simulink model "FieldOrientedController"  (R2020a)
settings: configuration reference "SLRT" (kept outside this file)
undefined symbols (not defined in the file): paramAdcAmperePerTransducerVolt, paramAdcTransducerVoltAtZeroAmpere, paramCurrentControlI, paramCurrentControlP, paramCurrentControlSatVoltage, paramEncoderCalibrationDuration, paramEncoderCalibrationMaxError, paramEncoderCalibrationVoltage, paramEncoderRotorPositionAtZeroCount, paramEncoderRotorPositionPerCount, paramOpenLoopVelocityAcceleration, paramOpenLoopVelocityToVoltsBias, paramOpenLoopVelocityToVoltsScalar, paramOverCurrentDuration, paramOverCurrentEnable, paramOverCurrentLimit, paramPwmCompareAtZeroVolt, paramPwmCompareMax, paramPwmComparePerVolt, paramVelocityControlI, paramVelocityControlP, paramVelocityControlSatCurrent, paramVelocityFilterCoeffDen, paramVelocityFilterCoeffNum, PolePairs, sampleTime
libraries: simulink x5
(part 1 of 2)
settings Model: DataDictionary=SGKitControllerData.sldd  EnableAccessToBaseWorkspace=off  OrderedModelArguments=off  Creator=The MathWorks, Inc.  LastModifiedBy=daniel.fonte
settings ConfigSetRef: SourceName=SLRT

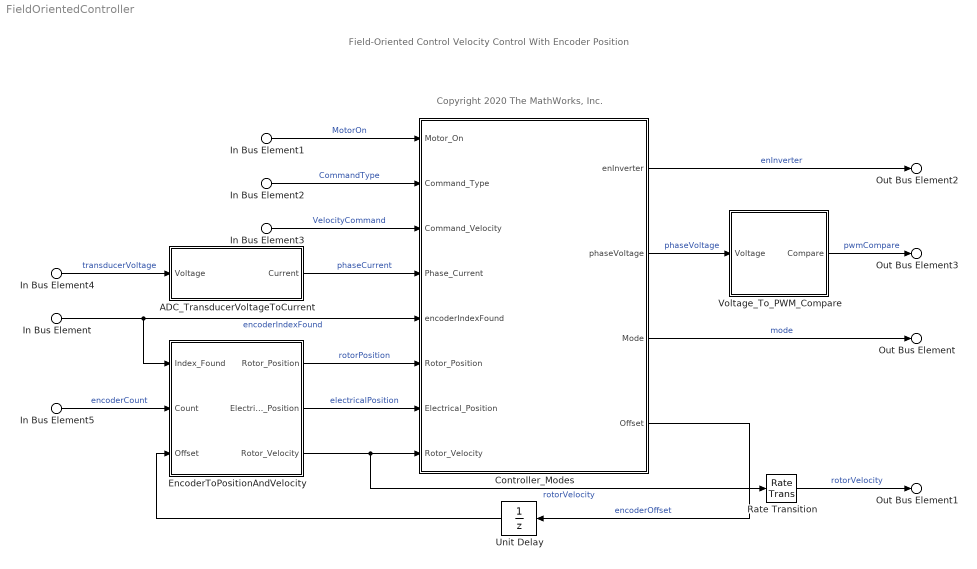
== system FieldOrientedController ==
  note: Field-Oriented Control
      | Velocity Control With Encoder Position
  note: Copyright 2020 The MathWorks, Inc.
  In Bus Element1 : Inport  PortName=userInputs  Element=motorOn
  In Bus Element2 : Inport  PortName=userInputs  Element=commandType
  In Bus Element3 : Inport  PortName=userInputs  Element=velocityCommand
  In Bus Element4 : Inport  Port=2  PortName=controllerFeedback  Element=transducerVoltage
  In Bus Element : Inport  Port=2  PortName=controllerFeedback  Element=encoderIndexFound
  In Bus Element5 : Inport  Port=2  PortName=controllerFeedback  Element=encoderCount
  ADC_TransducerVoltageToCurrent : Subsystem  VariantControl=kitType == 1
  Controller_Modes : Subsystem
  EncoderToPositionAndVelocity : Subsystem  VariantControl=ctrlVariantPosSns==PosSnsEnum.Encoder
  Rate Transition : RateTransition  OutPortSampleTime=sampleTime.VelocityControl
  Unit Delay : UnitDelay  InitialCondition=paramEncoderRotorPositionAtZeroCount  SampleTime=-1  StateName=encoderOffset  HasFrameUpgradeWarning=on
  Voltage_To_PWM_Compare : Subsystem
  Out Bus Element : Outport  PortName=controllerInfo  Element=mode
  Out Bus Element1 : Outport  PortName=controllerInfo  Element=rotorVelocity
  Out Bus Element2 : Outport  Port=2  PortName=motorCommands  Element=enInverter
  Out Bus Element3 : Outport  Port=2  PortName=motorCommands  Element=pwmCompare
  wires:
  EncoderToPositionAndVelocity/2(Electrical_Position) -> Controller_Modes/7(Electrical_Position)  "electricalPosition"
  EncoderToPositionAndVelocity/3(Rotor_Velocity) -> Rate Transition/1, Controller_Modes/8(Rotor_Velocity)  "rotorVelocity"
  Controller_Modes/4(Offset) -> Unit Delay/1  "encoderOffset"
  EncoderToPositionAndVelocity/1(Rotor_Position) -> Controller_Modes/6(Rotor_Position)  "rotorPosition"
  In Bus Element1/1 -> Controller_Modes/1(Motor_On)  "MotorOn"
  In Bus Element2/1 -> Controller_Modes/2(Command_Type)  "CommandType"
  In Bus Element3/1 -> Controller_Modes/3(Command_Velocity)  "VelocityCommand"
  In Bus Element/1 -> Controller_Modes/5(encoderIndexFound), EncoderToPositionAndVelocity/1(Index_Found)  "encoderIndexFound"
  Voltage_To_PWM_Compare/1(Compare) -> Out Bus Element3/1  "pwmCompare"
  In Bus Element5/1 -> EncoderToPositionAndVelocity/2(Count)  "encoderCount"
  Unit Delay/1 -> EncoderToPositionAndVelocity/3(Offset)
  In Bus Element4/1 -> ADC_TransducerVoltageToCurrent/1(Voltage)  "transducerVoltage"
  ADC_TransducerVoltageToCurrent/1(Current) -> Controller_Modes/4(Phase_Current)  "phaseCurrent"
  Controller_Modes/1(enInverter) -> Out Bus Element2/1  "enInverter"
  Controller_Modes/2(phaseVoltage) -> Voltage_To_PWM_Compare/1(Voltage)  "phaseVoltage"
  Controller_Modes/3(Mode) -> Out Bus Element/1  "mode"
  Rate Transition/1 -> Out Bus Element1/1  "rotorVelocity"

== system FieldOrientedController/ADC_TransducerVoltageToCurrent ==
  note: ADC Transducer Voltage to Current
  Voltage : Inport
  Add : Sum  Inputs=+-
  Bias_To_Remove : Constant  Value=paramAdcTransducerVoltAtZeroAmpere  OutDataTypeStr=Inherit: Inherit via back propagation  SampleTime=-1
  Product : Product
  Scalar : Constant  Value=paramAdcAmperePerTransducerVolt  OutDataTypeStr=Inherit: Inherit via back propagation  SampleTime=-1
  Current : Outport  VectorParamsAs1DForOutWhenUnconnected=off
  wires:
  Voltage/1 -> Add/1
  Scalar/1 -> Product/2
  Add/1 -> Product/1
  Bias_To_Remove/1 -> Add/2
  Product/1 -> Current/1  "PhaseCurrent"

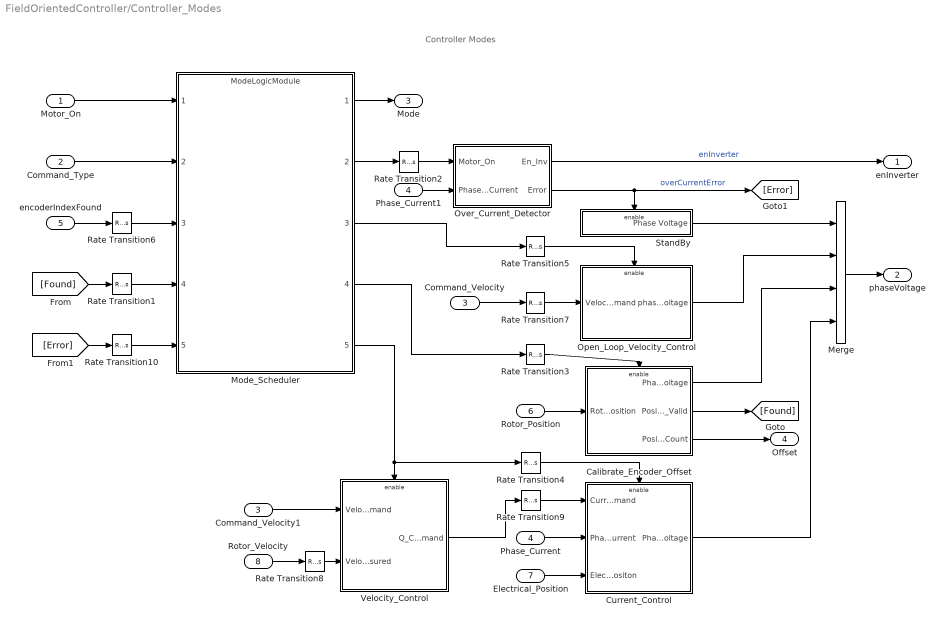
== system FieldOrientedController/Controller_Modes ==
  note: Controller Modes
  Motor_On : Inport
  Command_Type : Inport  Port=2
  Command_Velocity : Inport  Port=3
  Phase_Current : Inport  Port=4
  encoderIndexFound : Inport  Port=5
  Rotor_Position : Inport  Port=6
  Electrical_Position : Inport  Port=7
  Rotor_Velocity : Inport  Port=8
  Calibrate_Encoder_Offset : Subsystem
      mask Display: fprintf('Calibrate\nEncoder\nOffset')
  Command_Velocity1 : InportShadow  Port=3
  Current_Control : Subsystem
      mask Display: fprintf('Current\nControl')
  Merge : Merge  Inputs=4
      mask Display: fprintf(' ')
  Mode_Scheduler : ModelReference  ModelNameDialog=ModeLogicModule  SimulationMode=Normal  ModelReferenceVersion=1.378
  Open_Loop_Velocity_Control : Subsystem  TreatAsAtomicUnit=on
      settings: RTWFcnNameOpts=User specified  FunctionInterfaceSpec=Allow arguments (Optimized)
      mask Display: fprintf('Open Loop\nVelocity\nControl')
  Over_Current_Detector : Subsystem
      mask Display: %fprintf('Detect\nOvercurrent')
  Phase_Current1 : InportShadow  Port=4
  Rate Transition{1,6,8,10} (4 alike) : RateTransition  Integrity=off  OutPortSampleTime=sampleTime.VelocityControl
  Rate Transition{2..5,9} (5 alike) : RateTransition  Integrity=off
  Rate Transition7 : RateTransition  Integrity=off  OutPortSampleTime=sampleTime.CurrentControl
  StandBy : Subsystem  Description=Stand By mode for controller outputs constant phase voltages.  TreatAsAtomicUnit=on
      mask Display: fprintf('Disabled')
  Velocity_Control : Subsystem
      mask Display: fprintf('Velocity\nControl')
  enInverter : Outport  VectorParamsAs1DForOutWhenUnconnected=off
  phaseVoltage : Outport  Port=2  VectorParamsAs1DForOutWhenUnconnected=off
  Mode : Outport  Port=3  VectorParamsAs1DForOutWhenUnconnected=off
  Offset : Outport  Port=4  VectorParamsAs1DForOutWhenUnconnected=off
  wires:
  Rate Transition10/1 -> Mode_Scheduler/5
  [Error] -> Rate Transition10/1
  Calibrate_Encoder_Offset/2(Position_At_Zero_Count_Valid) -> [Found]
  Over_Current_Detector/2(Error) -> [Error], StandBy/Enable  "overCurrentError"
  Phase_Current1/1 -> Over_Current_Detector/2(Phase_Current)
  Rate Transition2/1 -> Over_Current_Detector/1(Motor_On)
  Mode_Scheduler/2 -> Rate Transition2/1
  Motor_On/1 -> Mode_Scheduler/1
  [Found] -> Rate Transition1/1
  Merge/1 -> phaseVoltage/1
  Command_Velocity/1 -> Rate Transition7/1
  Calibrate_Encoder_Offset/3(Position_At_Zero_Count) -> Offset/1
  Rotor_Position/1 -> Calibrate_Encoder_Offset/1(Rotor_Position)
  Calibrate_Encoder_Offset/1(Phase_Voltage) -> Merge/3
  StandBy/1(Phase Voltage) -> Merge/1
  Command_Type/1 -> Mode_Scheduler/2
  Mode_Scheduler/1 -> Mode/1
  Mode_Scheduler/4 -> Rate Transition3/1
  Rate Transition3/1 -> Calibrate_Encoder_Offset/Enable
  Rate Transition1/1 -> Mode_Scheduler/4
  Rate Transition7/1 -> Open_Loop_Velocity_Control/1(Velocity_Command)
  Open_Loop_Velocity_Control/1(phase_voltage) -> Merge/2
  Current_Control/1(Phase_Voltage) -> Merge/4
  Rate Transition4/1 -> Current_Control/Enable
  Rate Transition9/1 -> Current_Control/1(Current_Command)
  Velocity_Control/1(Q_Current_Command) -> Rate Transition9/1
  Mode_Scheduler/5 -> Rate Transition4/1, Velocity_Control/Enable
  Phase_Current/1 -> Current_Control/2(Phase_Current)
  Electrical_Position/1 -> Current_Control/3(Electrical_Positon)
  Rotor_Velocity/1 -> Rate Transition8/1
  Command_Velocity1/1 -> Velocity_Control/1(Velocity_Command)
  Rate Transition5/1 -> Open_Loop_Velocity_Control/Enable
  Mode_Scheduler/3 -> Rate Transition5/1
  encoderIndexFound/1 -> Rate Transition6/1
  Rate Transition8/1 -> Velocity_Control/2(Velocity_Measured)
  Over_Current_Detector/1(En_Inv) -> enInverter/1  "enInverter"
  Rate Transition6/1 -> Mode_Scheduler/3

== system FieldOrientedController/EncoderToPositionAndVelocity ==
  note: Quadrature Encoder To Position And Velocity
  Index_Found : Inport
  Count : Inport  Port=2
  Offset : Inport  Port=3
  Encoder_Count_To_Rotor_Position : Subsystem
  FilterTs15mS : DiscreteFilter  Numerator=paramVelocityFilterCoeffNum  Denominator=paramVelocityFilterCoeffDen  SampleTime=sampleTime.CurrentControl
  Position_Delta_To_Velocity : Subsystem  mask(Rotor position delta to velocity){positionDeltaBufferLength=8, sampleFrequency=1/sampleTime.EncoderPosition}
      mask prompts: positionDeltaBufferLength "Delay buffer length (must be power of two)"; sampleFrequency "Sample frequency (Hz)"
      mask help: Calculates velocity by summing the current position delta and a buffer of previous position deltas. Previous position deltas are stored in a circular buffer.
  Rotor_Position_Delta : Subsystem
  Rotor_To_Electrical_Position : Subsystem
      mask Display:
      | text(0.5, 0.5,...
      |   'E = mod(R*N_P_P,2\pi)',...
      |   'HorizontalAlignment', 'Center',...
      |   'VerticalAlignment', 'Middle',...
      |   'texmode', 'on')
  Rotor_Position : Outport  VectorParamsAs1DForOutWhenUnconnected=off
  Electrical_Position : Outport  Port=2  VectorParamsAs1DForOutWhenUnconnected=off
  Rotor_Velocity : Outport  Port=3  VectorParamsAs1DForOutWhenUnconnected=off
  wires:
  Rotor_Position_Delta/1(Position_Delta) -> Position_Delta_To_Velocity/1(Position_Delta)  "rotorPositionDelta"
  Offset/1 -> Encoder_Count_To_Rotor_Position/2(Position_At_Zero_Count), Rotor_Position_Delta/2(Encoder_Offset)
  Encoder_Count_To_Rotor_Position/1(Position) -> Rotor_Position_Delta/1(Rotor_Position), Rotor_To_Electrical_Position/1(R), Rotor_Position/1
  Rotor_To_Electrical_Position/1(E) -> Electrical_Position/1
  Count/1 -> Encoder_Count_To_Rotor_Position/1(Count)
  Index_Found/1 -> Rotor_Position_Delta/3(Encoder_Index_Found)
  Position_Delta_To_Velocity/1(Velocity) -> FilterTs15mS/1
  FilterTs15mS/1 -> Rotor_Velocity/1

== system FieldOrientedController/Voltage_To_PWM_Compare ==
  note: Voltage To PWM Compare
  Voltage : Inport
  Add : Sum  OutDataTypeStr=Inherit: Inherit via back propagation
  Bias : Constant  Value=paramPwmCompareAtZeroVolt  OutDataTypeStr=Inherit: Inherit via back propagation  SampleTime=-1
  Data_Type_Conversion : DataTypeConversion  OutDataTypeStr=uint16  LockScale=on
  Saturation : Saturate  UpperLimit=paramPwmCompareMax  LowerLimit=0
      settings: AttributesFormatString=|
      | --------------------------------
      | Upper Limit = %<UpperLimit>
      | Lower Limit = %<LowerLimit>
  Slope : Gain  Gain=paramPwmComparePerVolt
      settings: AttributesFormatString=|
      | ----------------------------------------
      | Gain = %<Gain>
  Compare : Outport  VectorParamsAs1DForOutWhenUnconnected=off
  wires:
  Add/1 -> Saturation/1
  Bias/1 -> Add/2
  Saturation/1 -> Data_Type_Conversion/1
  Slope/1 -> Add/1
  Voltage/1 -> Slope/1  "phaseVoltage"
  Data_Type_Conversion/1 -> Compare/1  "pwmCompare"

== system FieldOrientedController/Controller_Modes/Calibrate_Encoder_Offset ==
  note: Calibrate Encoder Offset
  Rotor_Position : Inport  PortDimensions=1  Interpolate=off
  Enable : EnablePort  StatesWhenEnabling=reset
      settings: AttributesFormatString=|
      | ----------------------------------------
      | States when enabling = %<StatesWhenEnabling>
  Encoder_Calibration : Subsystem
  Phase_Voltage : Outport  PortDimensions=3  InitialOutput=0  VectorParamsAs1DForOutWhenUnconnected=off
  Position_At_Zero_Count_Valid : Outport  Port=2  InitialOutput=0  VectorParamsAs1DForOutWhenUnconnected=off
  Position_At_Zero_Count : Outport  Port=3  InitialOutput=paramEncoderRotorPositionAtZeroCount  VectorParamsAs1DForOutWhenUnconnected=off
      settings: AttributesFormatString=|
      | ---------------------------------
      | Initial Output = %<InitialOutput>
  wires:
  Encoder_Calibration/2(Position_Valid) -> Position_At_Zero_Count_Valid/1
  Encoder_Calibration/1(Phase_Voltage) -> Phase_Voltage/1
  Rotor_Position/1 -> Encoder_Calibration/1(Rotor_Position)
  Encoder_Calibration/3(Position_At_Zero_Count) -> Position_At_Zero_Count/1

== system FieldOrientedController/Controller_Modes/Current_Control ==
  note: Current Control
  Current_Command : Inport
  Phase_Current : Inport  Port=2
  Electrical_Positon : Inport  Port=3
  Enable : EnablePort  StatesWhenEnabling=reset
      settings: AttributesFormatString=|
      | ----------------------------------------
      | States when enabling = %<StatesWhenEnabling>
  FOC_Current_Control : Subsystem
  Phase_Voltage : Outport  VectorParamsAs1DForOutWhenUnconnected=off
  wires:
  Electrical_Positon/1 -> FOC_Current_Control/3(Electrical_Position)
  FOC_Current_Control/1(Phase_Voltage) -> Phase_Voltage/1
  Current_Command/1 -> FOC_Current_Control/1(Current_Command)
  Phase_Current/1 -> FOC_Current_Control/2(Phase_Current)

== system FieldOrientedController/Controller_Modes/Open_Loop_Velocity_Control ==
  note: Open Loop Velocity Control
  Velocity_Command : Inport
  Enable : EnablePort  StatesWhenEnabling=reset
      settings: AttributesFormatString=|
      | ----------------------------------------
      | States when enabling = %<StatesWhenEnabling>
  Open_Loop_Velocity_Control : Subsystem
  Signal Conversion : SignalConversion  OverrideOpt=off
  phase_voltage : Outport  VectorParamsAs1DForOutWhenUnconnected=off
  wires:
  Open_Loop_Velocity_Control/1(Phase_Voltage) -> Signal Conversion/1  "phaseVoltage"
  Velocity_Command/1 -> Open_Loop_Velocity_Control/1(Velocity_Command)
  Signal Conversion/1 -> phase_voltage/1

== system FieldOrientedController/Controller_Modes/Over_Current_Detector ==
  note: Over Current Detector
  Motor_On : Inport
  Phase_Current : Inport  Port=2
  AND : Logic  IconShape=distinctive  AllPortsSameDT=off  OutDataTypeStr=boolean
  AND1 : Logic  IconShape=distinctive  AllPortsSameDT=off  OutDataTypeStr=boolean
  Abs : Abs
  Demux : Demux  Outputs=2
  Detect_Over_Current_Error : Stateflow chart  TreatAsAtomicUnit=on
  Enable_Over_Current_Detection : Constant  Value=paramOverCurrentEnable  OutDataTypeStr=Inherit: Inherit via back propagation
  Motor_On1 : InportShadow
  NOT : Logic  Operator=NOT  IconShape=distinctive  AllPortsSameDT=off  OutDataTypeStr=boolean
  En_Inv : Outport  VectorParamsAs1DForOutWhenUnconnected=off
  Error : Outport  Port=2  VectorParamsAs1DForOutWhenUnconnected=off
  wires:
  Enable_Over_Current_Detection/1 -> AND/2
  AND/1 -> Detect_Over_Current_Error/1(enableOverCurrentDetect)
  Motor_On1/1 -> AND1/1
  NOT/1 -> AND1/2
  AND1/1 -> En_Inv/1  "enableInverter"
  Motor_On/1 -> AND/1
  Demux/1 -> Detect_Over_Current_Error/2(phaseCurrentA)
  Detect_Over_Current_Error/1(error) -> NOT/1, Error/1  "overCurrentErrorDetected"
  Demux/2 -> Detect_Over_Current_Error/3(phaseCurrentB)
  Abs/1 -> Demux/1
  Phase_Current/1 -> Abs/1

== system FieldOrientedController/Controller_Modes/StandBy ==
  note: Disabled
  Enable : EnablePort
      settings: AttributesFormatString=|
      | ----------------------------------------
      | States when enabling = %<StatesWhenEnabling>
  Constant : Constant  Value=[0 0 0]  OutDataTypeStr=Inherit: Inherit via back propagation
  Phase Voltage : Outport  InitialOutput=[0 0 0]  VectorParamsAs1DForOutWhenUnconnected=off
      settings: AttributesFormatString=--------------------------------------------\nInitial Output = %<InitialOutput>
  wires:
  Constant/1 -> Phase Voltage/1

== system FieldOrientedController/Controller_Modes/Velocity_Control ==
  note: Velocity Control
  Velocity_Command : Inport
  Velocity_Measured : Inport  Port=2
  Enable : EnablePort  StatesWhenEnabling=reset
      settings: AttributesFormatString=|
      | ----------------------------------------
      | States when enabling = %<StatesWhenEnabling>
  Subtract : Sum  Inputs=+-
  Velocity_PID_Controller : simulink/Continuous/PID Controller  Controller=PI  Form=Parallel  TimeDomain=Discrete-time  UseExternalTs=off  SampleTime=sampleTime.VelocityControl  IntegratorMethod=Forward Euler  FilterMethod=Forward Euler  ControllerParametersSource=internal  P=paramVelocityControlP  I=paramVelocityControlI  D=0  UseFilter=on  N=0  TunerSelectOption=Transfer Function Based (PID Tuner App)  InitialConditionSource=internal  InitialConditionForIntegrator=0  InitialConditionForFilter=0  DifferentiatorICPrevScaledInput=0  ExternalReset=none  TrackingMode=off  Kt=1  LimitOutput=on  UpperSaturationLimit=paramVelocityControlSatCurrent  LowerSaturationLimit=-paramVelocityControlSatCurrent  LinearizeAsGain=off  AntiWindupMode=clamping  Kb=1  POutMin=[]  POutMax=[]  IOutMin=[]  IOutMax=[]  DOutMin=[]  DOutMax=[]  NOutMin=[]  NOutMax=[]  SumOutMin=[]  SumOutMax=[]  SaturationOutMin=[]  SaturationOutMax=[]  PParamMin=[]  PParamMax=[]  IParamMin=[]  IParamMax=[]  DParamMin=[]  DParamMax=[]  NParamMin=[]  NParamMax=[]  KbParamMin=[]  KbParamMax=[]  KtParamMin=[]  KtParamMax=[]  KbOutMin=[]  KbOutMax=[]  KtOutMin=[]  KtOutMax=[]  IntegratorOutMin=[]  IntegratorOutMax=[]  FilterOutMin=[]  FilterOutMax=[]  SumI1OutMin=[]  SumI1OutMax=[]  SumI2OutMin=[]  SumI2OutMax=[]  SumI3OutMin=[]  SumI3OutMax=[]  SumI4OutMin=[]  SumI4OutMax=[]  SumDOutMin=[]  SumDOutMax=[]  DifferentiatorOutMin=[]  DifferentiatorOutMax=[]  FilterDiffOutCoefMin=[]  FilterDiffOutCoefMax=[]  ReciprocalOutMin=[]  ReciprocalOutMax=[]  SumDenOutMin=[]  SumDenOutMax=[]  SumNumOutMin=[]  SumNumOutMax=[]  DivideOutMin=[]  DivideOutMax=[]  UdiffTsProdOutMin=[]  UdiffTsProdOutMax=[]  NTsProdOutMin=[]  NTsProdOutMax=[]  UintegralTsProdOutMin=[]  UintegralTsProdOutMax=[]  UngainTsProdOutMin=[]  UngainTsProdOutMax=[]  IntegratorContinuousStateAttributes=''  IntegratorStateMustResolveToSignalObject=off  IntegratorRTWStateStorageClass=Auto  FilterContinuousStateAttributes=''  FilterStateMustResolveToSignalObject=off  FilterRTWStateStorageClass=Auto  ParallelPVariant=InternalParameters  IdealPVariant=Disabled  IVariant=InternalParameters  DVariant=Disabled  IntegratorVariant=Discrete  SatVariant=Enabled  AWVariant=DiscClampingParallel  PCopyVariant=Disabled  TRVariant=Disabled  FdbkBlocksVariant=Forward  IdealPFdbkVariant=Disabled  SatFdbkVariant=Disabled  DerivativeFilterVariant=Disabled  NVariant=Disabled  NCopyVariant=Disabled_SignalSpec  FilterICVariant=Disabled  IntegratorICVariant=InternalICs  ExternalResetVariant=Disabled  TRSumVariant=Passthrough  SumFdbkVariant=Disabled  SumVariant=Sum_PI  TsampFilterVariant=InternalTs  TsampNgainVariant=Passthrough  TsampIntegralVariant=Passthrough
  Q_Current_Command : Outport  InitialOutput=0  VectorParamsAs1DForOutWhenUnconnected=off
  wires:
  Velocity_Command/1 -> Subtract/1
  Velocity_Measured/1 -> Subtract/2
  Velocity_PID_Controller/1 -> Q_Current_Command/1  "qCurrentCommand"
  Subtract/1 -> Velocity_PID_Controller/1

== system FieldOrientedController/EncoderToPositionAndVelocity/Encoder_Count_To_Rotor_Position ==
  note: Encoder Count To Rotor Position
  Count : Inport
  Position_At_Zero_Count : Inport  Port=2
  Add : Sum  AccumDataTypeStr=single
  Data_Type_Convert : DataTypeConversion  OutDataTypeStr=single
  Mod_Two_Pi_Once : Subsystem
      mask Display:
      | text(0.5, 0.5,'Mod 2\pi',...
      |   'HorizontalAlignment', 'Center',...
      |   'VerticalAlignment', 'Middle',...
      |   'texmode', 'on')
  Rotor_Position_Per_Count : Gain  Gain=paramEncoderRotorPositionPerCount  ParamDataTypeStr=single  OutDataTypeStr=single
      settings: AttributesFormatString=|
      | ------------------------------------------------
      | Gain = %<Gain>
  Position : Outport  VectorParamsAs1DForOutWhenUnconnected=off
  wires:
  Count/1 -> Data_Type_Convert/1
  Mod_Two_Pi_Once/1(Mod_X_Two_Pi) -> Position/1  "rotorPosition"
  Add/1 -> Mod_Two_Pi_Once/1(X)
  Rotor_Position_Per_Count/1 -> Add/1
  Position_At_Zero_Count/1 -> Add/2
  Data_Type_Convert/1 -> Rotor_Position_Per_Count/1

== system FieldOrientedController/EncoderToPositionAndVelocity/Position_Delta_To_Velocity ==
  note: Rotor Position Delta To Velocity
  Position_Delta : Inport  SampleTime=sampleTime.EncoderPosition
  Rotor_Position_Delta_To_Velocity : MATLAB Function  TreatAsAtomicUnit=on
  Velocity : Outport  SampleTime=sampleTime.EncoderPosition  VectorParamsAs1DForOutWhenUnconnected=off
  wires:
  Rotor_Position_Delta_To_Velocity/1(rotorVelocity) -> Velocity/1
  Position_Delta/1 -> Rotor_Position_Delta_To_Velocity/1(positionDelta)

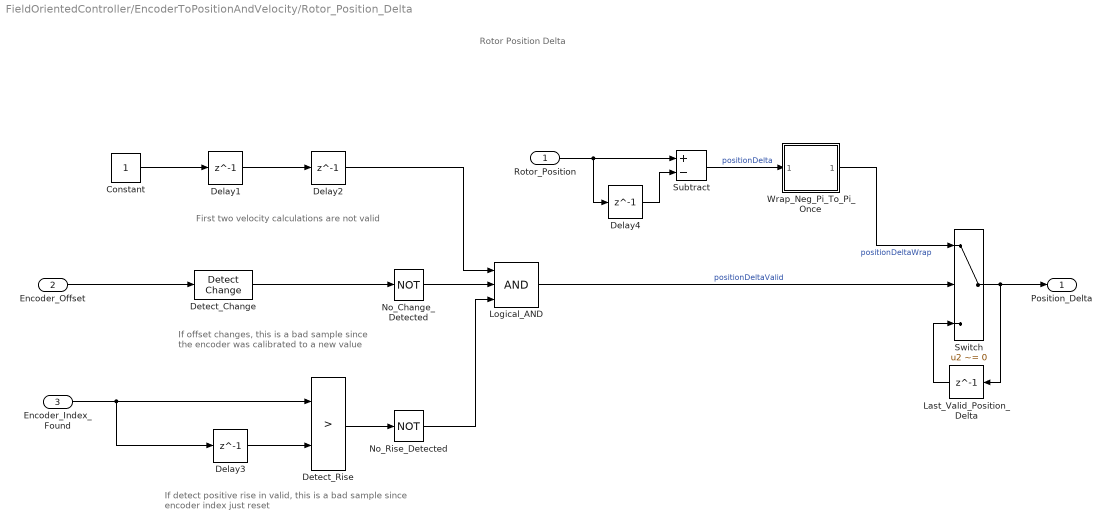
== system FieldOrientedController/EncoderToPositionAndVelocity/Rotor_Position_Delta ==
  note: If offset changes, this is a bad sample since
      | the encoder was calibrated to a new value
  note: First two velocity calculations are not valid
  note: If detect positive rise in valid, this is a bad sample since
      | encoder index just reset
  note: Rotor Position Delta
  Rotor_Position : Inport  SampleTime=sampleTime.EncoderPosition
  Encoder_Offset : Inport  Port=2  SampleTime=sampleTime.EncoderPosition
  Encoder_Index_Found : Inport  Port=3  SampleTime=sampleTime.EncoderPosition
  Constant : Constant  OutDataTypeStr=Inherit: Inherit via back propagation  SampleTime=-1
  Delay{1..4} (4 alike) : Delay  DelayLength=1
  Detect_Change : simulink/Logic and Bit Operations/Detect Change  vinit=0  OutDataTypeStr=boolean
  Detect_Rise : RelationalOperator  Operator=>  OutDataTypeStr=boolean  ZeroCross=off  RndMeth=Nearest
  Last_Valid_Position_Delta : Delay  DelayLength=1
  Logical_AND : Logic  Inputs=3  IconShape=distinctive  AllPortsSameDT=off  OutDataTypeStr=boolean
  No_Change_Detected : Logic  Operator=NOT  IconShape=distinctive  AllPortsSameDT=off  OutDataTypeStr=boolean
  No_Rise_Detected : Logic  Operator=NOT  IconShape=distinctive  AllPortsSameDT=off  OutDataTypeStr=boolean
  Subtract : Sum  Inputs=+-  InputSameDT=on
  Switch : Switch  Criteria=u2 ~= 0  InputSameDT=on
  Wrap_Neg_Pi_To_Pi_Once : Subsystem
      mask Display:
      | text(0.5, 0.5,['  Wrap' sprintf('\n') '-\pi to \pi'],...
      |   'HorizontalAlignment', 'Center',...
      |   'VerticalAlignment', 'Middle',...
      |   'texmode', 'on');
  Position_Delta : Outport  VectorParamsAs1DForOutWhenUnconnected=off
  wires:
  No_Change_Detected/1 -> Logical_AND/2
  Detect_Change/1 -> No_Change_Detected/1
  Encoder_Offset/1 -> Detect_Change/1
  Wrap_Neg_Pi_To_Pi_Once/1(Wrap) -> Switch/1  "positionDeltaWrap"
  Encoder_Index_Found/1 -> Detect_Rise/1, Delay3/1
  Rotor_Position/1 -> Subtract/1, Delay4/1
  Subtract/1 -> Wrap_Neg_Pi_To_Pi_Once/1(Position)  "positionDelta"
  Delay2/1 -> Logical_AND/1
  Delay4/1 -> Subtract/2
  Logical_AND/1 -> Switch/2  "positionDeltaValid"
  Delay3/1 -> Detect_Rise/2
  Last_Valid_Position_Delta/1 -> Switch/3
  Detect_Rise/1 -> No_Rise_Detected/1
  No_Rise_Detected/1 -> Logical_AND/3
  Switch/1 -> Position_Delta/1, Last_Valid_Position_Delta/1
  Constant/1 -> Delay1/1
  Delay1/1 -> Delay2/1

== system FieldOrientedController/EncoderToPositionAndVelocity/Rotor_To_Electrical_Position ==
  note: Rotor To Electrical Position
  R : Inport
  Gain : Gain  Gain=PolePairs  OutDataTypeStr=Inherit: Same as input
      settings: AttributesFormatString=|
      | -------------------------------
      | Gain = %<Gain>
  Mod_Two_Pi : Subsystem
      mask Display:
      | text(0.5, 0.5,'Mod 2\pi',...
      |   'HorizontalAlignment', 'Center',...
      |   'VerticalAlignment', 'Middle',...
      |   'texmode', 'on')
  E : Outport  VectorParamsAs1DForOutWhenUnconnected=off
  wires:
  Gain/1 -> Mod_Two_Pi/1(X)
  Mod_Two_Pi/1(Mod_X_Two_Pi) -> E/1
  R/1 -> Gain/1

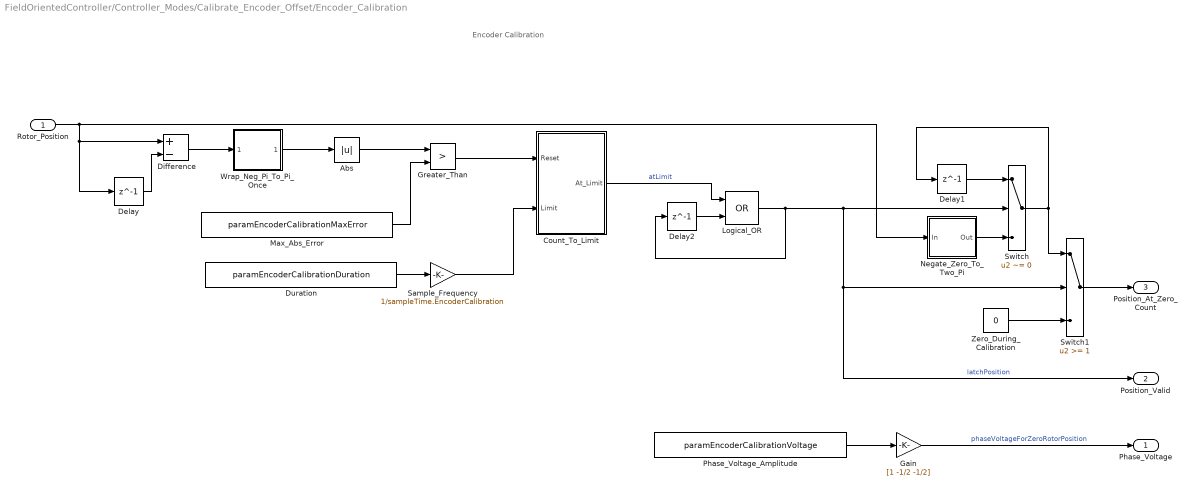
== system FieldOrientedController/Controller_Modes/Calibrate_Encoder_Offset/Encoder_Calibration ==
  note: Encoder Calibration
  Rotor_Position : Inport  OutMin=0  OutMax=2*pi  PortDimensions=1  SampleTime=sampleTime.EncoderCalibration  Interpolate=off
  Abs : Abs
  Count_To_Limit : Subsystem
  Delay : Delay  DelayLength=1
  Delay1 : Delay  DelayLength=1  InitialCondition=0
  Delay2 : Delay  DelayLength=1  InitialCondition=0
  Difference : Sum  Inputs=+-
  Duration : Constant  Value=paramEncoderCalibrationDuration  OutDataTypeStr=Inherit: Inherit via back propagation  SampleTime=-1
  Gain : Gain  Gain=[1 -1/2 -1/2]
      settings: AttributesFormatString=|
      | ----------------------------------
      | Gain = %<Gain>
  Greater_Than : RelationalOperator  Operator=>  OutDataTypeStr=boolean  RndMeth=Nearest
  Logical_OR : Logic  Operator=OR  IconShape=distinctive  AllPortsSameDT=off  OutDataTypeStr=boolean
  Max_Abs_Error : Constant  Value=paramEncoderCalibrationMaxError  OutDataTypeStr=Inherit: Inherit via back propagation  SampleTime=-1
  Negate_Zero_To_Two_Pi : Subsystem
      mask Display:
      | text(0.5, 0.5,['Negate' sprintf('\n') '0 to 2\pi'],...
      |   'HorizontalAlignment', 'Center',...
      |   'VerticalAlignment', 'Middle',...
      |   'texmode', 'on');
  Phase_Voltage_Amplitude : Constant  Value=paramEncoderCalibrationVoltage  OutDataTypeStr=Inherit: Inherit via back propagation  SampleTime=-1
  Sample_Frequency : Gain  Gain=1/sampleTime.EncoderCalibration
      settings: AttributesFormatString=|
      | ----------------------------------
      | Gain = %<Gain>
  Switch : Switch  Criteria=u2 ~= 0  Threshold=1
  Switch1 : Switch  Threshold=1
  Wrap_Neg_Pi_To_Pi_Once : Subsystem
      mask Display:
      | text(0.5, 0.5,['  Wrap' sprintf('\n') '-\pi to \pi'],...
      |   'HorizontalAlignment', 'Center',...
      |   'VerticalAlignment', 'Middle',...
      |   'texmode', 'on');
  Zero_During_Calibration : Constant  Value=0  OutDataTypeStr=Inherit: Inherit via back propagation
  Phase_Voltage : Outport  VectorParamsAs1DForOutWhenUnconnected=off
  Position_Valid : Outport  Port=2  VectorParamsAs1DForOutWhenUnconnected=off
  Position_At_Zero_Count : Outport  Port=3  VectorParamsAs1DForOutWhenUnconnected=off
  wires:
  Delay2/1 -> Logical_OR/2
  Count_To_Limit/1(At_Limit) -> Logical_OR/1  "atLimit"
  Sample_Frequency/1 -> Count_To_Limit/2(Limit)
  Negate_Zero_To_Two_Pi/1(Out) -> Switch/3
  Delay1/1 -> Switch/1
  Rotor_Position/1 -> Delay/1, Difference/1, Negate_Zero_To_Two_Pi/1(In)
  Delay/1 -> Difference/2
  Switch/1 -> Delay1/1, Switch1/1
  Logical_OR/1 -> Switch/2, Switch1/2, Position_Valid/1, Delay2/1  "latchPosition"
  Zero_During_Calibration/1 -> Switch1/3
  Max_Abs_Error/1 -> Greater_Than/2
  Abs/1 -> Greater_Than/1
  Switch1/1 -> Position_At_Zero_Count/1
  Wrap_Neg_Pi_To_Pi_Once/1(Wrap) -> Abs/1
  Difference/1 -> Wrap_Neg_Pi_To_Pi_Once/1(Position)
  Duration/1 -> Sample_Frequency/1
  Phase_Voltage_Amplitude/1 -> Gain/1
  Gain/1 -> Phase_Voltage/1  "phaseVoltageForZeroRotorPosition"
  Greater_Than/1 -> Count_To_Limit/1(Reset)

== system FieldOrientedController/Controller_Modes/Current_Control/FOC_Current_Control ==
  note: FOC Current Control
  note: Copyright 2020 The MathWorks, Inc.
  Current_Command : Inport
  Phase_Current : Inport  Port=2
  Electrical_Position : Inport  Port=3
  Clarke_Transform : Subsystem
      mask Display:
      | port_label('input',1,'ABC')
      | port_label('output',1,'\alpha','texmode', 'on')
      | port_label('output',2,'\beta','texmode', 'on')
  DQ_Current_Control : Subsystem
  Inverse_Clarke_Transform : Subsystem  VariantControl=INVERSE_CLARKE_TRANSFORM
      mask Display:
      | port_label('input',1,'\alpha','texmode', 'on')
      | port_label('input',2,'\beta','texmode', 'on')
      | port_label('output',1,'a')
      | port_label('output',2,'b')
      | port_label('output',3,'c')
  Inverse_Park_Transform : Subsystem
      mask Display:
      | port_label('input',1,'D')
      | port_label('input',2,'Q')
      | port_label('input',3,'Sin')
      | port_label('input',4,'Cos')
      | port_label('output',1,'\alpha','texmode', 'on')
      | port_label('output',2,'\beta','texmode', 'on')
  Mux : Mux  Inputs=3
  Park_Transform : Subsystem
      mask Display:
      | port_label('input',1,'\alpha','texmode', 'on')
      | port_label('input',2,'\beta','texmode', 'on')
      | port_label('input',3,'Sin')
      | port_label('input',4,'Cos')
      | port_label('output',1,'D')
      | port_label('output',2,'Q')
  Sine_Cosine : Trigonometry  Operator=sincos
  Space_Vector_Modulation1 : Subsystem  VariantControl=SpaceVectorModulation_JB
      mask Display:
      | plot([0.000 0.020 0.041 0.061 0.082 0.102 0.122 0.143 0.163 0.184 0.204 0.224 0.245 0.265 0.286 0.306 0.327 0.347 0.367 0.388 0.408 0.429 0.449 0.469 0.490 0.510 0.531 0.551 0.571 0.592 0.612 0.633 0.653 0.673 0.694 0.714 0.735 0.755 0.776 0.796 0.816 0.837 0.857 0.878 0.898 0.918 0.939 0.959 0.980 1.000 ], ...
      |      [0.500 0.586 0.671 0.753 0.831 0.858 0.875 0.885 0.890 0.887 0.879 0.864 0.844 0.855 0.872 0.884 0.889 0.888 0.881 0.867 0.847 0.793 0.713 0.629 0.543 0.457 0.371 0.287 0.207 0.153 0.133 0.119 0.112 0.111 0.116 0.128 0.145 0.156 0.136 0.121 0.113 0.110 0.115 0.125 0.142 0.169 0.247 0.329 0.414 0.500 ])
  Phase_Voltage : Outport  VectorParamsAs1DForOutWhenUnconnected=off
  wires:
  Sine_Cosine/1 -> Inverse_Park_Transform/3(Sin_Coefficient), Park_Transform/3(Sin_Coefficient)  "sinCoefficient"
  Sine_Cosine/2 -> Inverse_Park_Transform/4(Cos_Coefficient), Park_Transform/4(Cos_Coefficient)  "cosCoefficient"
  Mux/1 -> Space_Vector_Modulation1/1(ABC)  "abcVoltage"
  Electrical_Position/1 -> Sine_Cosine/1
  Space_Vector_Modulation1/1(ABC_SVM) -> Phase_Voltage/1  "svmVoltage"
  Phase_Current/1 -> Clarke_Transform/1(ABC)
  Clarke_Transform/1(Alpha) -> Park_Transform/1(Alpha)  "alphaCurrent"
  Clarke_Transform/2(Beta) -> Park_Transform/2(Beta)  "betaCurrent"
  Inverse_Park_Transform/1(Alpha) -> Inverse_Clarke_Transform/1(Alpha)  "alphaVoltage"
  Inverse_Park_Transform/2(Beta) -> Inverse_Clarke_Transform/2(Beta)  "betaVoltage"
  Park_Transform/1(D) -> DQ_Current_Control/2(D_Current)  "dCurrent"
  Park_Transform/2(Q) -> DQ_Current_Control/3(Q_Current)  "qCurrent"
  Current_Command/1 -> DQ_Current_Control/1(Q_Command)
  DQ_Current_Control/1(D_Voltage) -> Inverse_Park_Transform/1(D)  "dVoltage"
  DQ_Current_Control/2(Q_Voltage) -> Inverse_Park_Transform/2(Q)  "qVoltage"
  Inverse_Clarke_Transform/2(b) -> Mux/2
  Inverse_Clarke_Transform/1(a) -> Mux/1
  Inverse_Clarke_Transform/3(b1) -> Mux/3

== system FieldOrientedController/Controller_Modes/Open_Loop_Velocity_Control/Open_Loop_Velocity_Control ==
  note: Open Loop Velocity Control
  Velocity_Command : Inport  SampleTime=sampleTime.OpenLoopVelocityControl
  Direct_Voltage : Constant  Value=0  OutDataTypeStr=Inherit: Inherit via back propagation
  Electrical_Velocity_To_Position : Subsystem
  Inverse_Clarke_Transform1 : Subsystem  VariantControl=INVERSE_CLARKE_TRANSFORM
      mask Display:
      | port_label('input',1,'\alpha','texmode', 'on')
      | port_label('input',2,'\beta','texmode', 'on')
      | port_label('output',1,'a')
      | port_label('output',2,'b')
      | port_label('output',3,'c')
  Inverse_Park_Transform : Subsystem
      mask Display:
      | port_label('input',1,'D')
      | port_label('input',2,'Q')
      | port_label('input',3,'Sin')
      | port_label('input',4,'Cos')
      | port_label('output',1,'\alpha','texmode', 'on')
      | port_label('output',2,'\beta','texmode', 'on')
  Mux : Mux  Inputs=3
  Ramp_Velocity : Subsystem
  Rotor_Velocity_To_Volts : Subsystem
  Sine_Cosine : Trigonometry  Operator=sincos
  Phase_Voltage : Outport  VectorParamsAs1DForOutWhenUnconnected=off
  wires:
  Electrical_Velocity_To_Position/1(EP) -> Sine_Cosine/1
  Ramp_Velocity/2(Electrical_Velocity) -> Electrical_Velocity_To_Position/1(EV)
  Ramp_Velocity/1(Rotor_Velocity) -> Rotor_Velocity_To_Volts/1(RV)
  Direct_Voltage/1 -> Inverse_Park_Transform/1(D)
  Velocity_Command/1 -> Ramp_Velocity/1(Velocity_Command)
  Mux/1 -> Phase_Voltage/1
  Sine_Cosine/1 -> Inverse_Park_Transform/3(Sin_Coefficient)
  Sine_Cosine/2 -> Inverse_Park_Transform/4(Cos_Coefficient)
  Rotor_Velocity_To_Volts/1(V) -> Inverse_Park_Transform/2(Q)  "quadratureVoltage"
  Inverse_Clarke_Transform1/1(a) -> Mux/1
  Inverse_Clarke_Transform1/2(b) -> Mux/2
  Inverse_Clarke_Transform1/3(b1) -> Mux/3
  Inverse_Park_Transform/1(Alpha) -> Inverse_Clarke_Transform1/1(Alpha)
  Inverse_Park_Transform/2(Beta) -> Inverse_Clarke_Transform1/2(Beta)

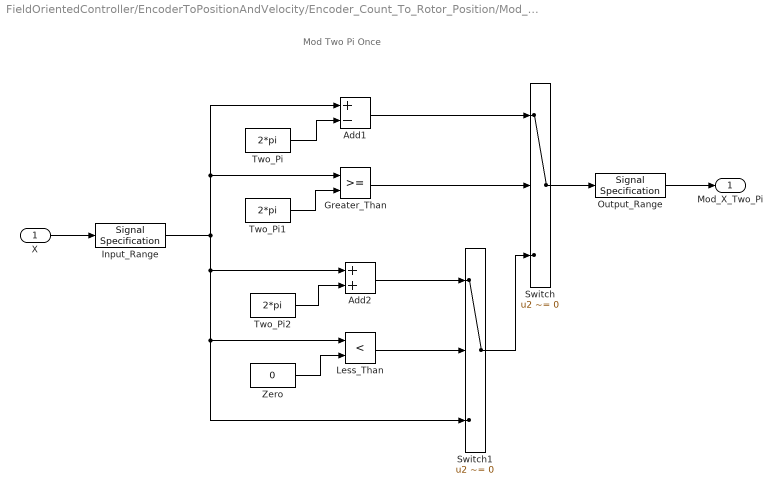
== system FieldOrientedController/EncoderToPositionAndVelocity/Encoder_Count_To_Rotor_Position/Mod_Two_Pi_Once ==
  note: Mod Two Pi Once
  X : Inport
  Add1 : Sum  Inputs=+-
  Add2 : Sum
  Greater_Than : RelationalOperator  OutDataTypeStr=boolean  RndMeth=Nearest
  Input_Range : SignalSpecification  OutMin=-4*pi  OutMax=4*pi
      settings: AttributesFormatString=|
      | -----------------------
      | Min = %<OutMin>
      | Max = %<OutMax>
  Less_Than : RelationalOperator  Operator=<  OutDataTypeStr=boolean  RndMeth=Nearest
  Output_Range : SignalSpecification  OutMin=0  OutMax=2*pi
      settings: AttributesFormatString=|
      | -----------------------
      | Min = %<OutMin>
      | Max = %<OutMax>
  Switch : Switch  Criteria=u2 ~= 0  InputSameDT=on
  Switch1 : Switch  Criteria=u2 ~= 0  InputSameDT=on
  Two_Pi : Constant  Value=2*pi  OutDataTypeStr=Inherit: Inherit via back propagation
  Two_Pi1 : Constant  Value=2*pi  OutDataTypeStr=Inherit: Inherit via back propagation
  Two_Pi2 : Constant  Value=2*pi  OutDataTypeStr=Inherit: Inherit via back propagation
  Zero : Constant  Value=0  OutDataTypeStr=Inherit: Inherit via back propagation
  Mod_X_Two_Pi : Outport  VectorParamsAs1DForOutWhenUnconnected=off
  wires:
  Output_Range/1 -> Mod_X_Two_Pi/1
  Zero/1 -> Less_Than/2
  Two_Pi2/1 -> Add2/2
  Add2/1 -> Switch1/1
  Less_Than/1 -> Switch1/2
  Switch1/1 -> Switch/3
  Two_Pi1/1 -> Greater_Than/2
  Two_Pi/1 -> Add1/2
  Add1/1 -> Switch/1
  Greater_Than/1 -> Switch/2
  X/1 -> Input_Range/1
  Switch/1 -> Output_Range/1
  Input_Range/1 -> Add1/1, Greater_Than/1, Add2/1, Less_Than/1, Switch1/3

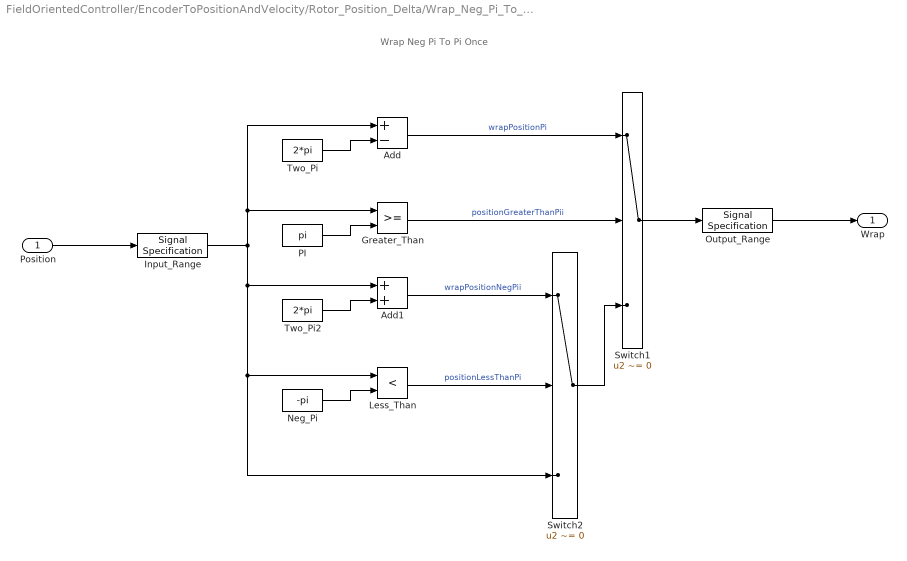
== system FieldOrientedController/EncoderToPositionAndVelocity/Rotor_Position_Delta/Wrap_Neg_Pi_To_Pi_Once ==
  note: Wrap Neg Pi To Pi Once
  Position : Inport
  Add : Sum  Inputs=+-  OutDataTypeStr=Inherit: Inherit via back propagation
  Add1 : Sum
  Greater_Than : RelationalOperator  OutDataTypeStr=boolean  RndMeth=Nearest
  Input_Range : SignalSpecification  OutMin=-4*pi  OutMax=4*pi
      settings: AttributesFormatString=|
      | -----------------------
      | Min = %<OutMin>
      | Max = %<OutMax>
  Less_Than : RelationalOperator  Operator=<  OutDataTypeStr=boolean  RndMeth=Nearest
  Neg_Pi : Constant  Value=-pi  OutDataTypeStr=Inherit: Inherit via back propagation
  Output_Range : SignalSpecification  OutMin=-pi  OutMax=pi
      settings: AttributesFormatString=|
      | -----------------------
      | Min = %<OutMin>
      | Max = %<OutMax>
  PI : Constant  Value=pi  OutDataTypeStr=Inherit: Inherit via back propagation
  Switch1 : Switch  Criteria=u2 ~= 0
  Switch2 : Switch  Criteria=u2 ~= 0
  Two_Pi : Constant  Value=2*pi  OutDataTypeStr=Inherit: Inherit via back propagation
  Two_Pi2 : Constant  Value=2*pi  OutDataTypeStr=Inherit: Inherit via back propagation
  Wrap : Outport  VectorParamsAs1DForOutWhenUnconnected=off
  wires:
  Input_Range/1 -> Greater_Than/1, Add/1, Add1/1, Switch2/3, Less_Than/1
  Output_Range/1 -> Wrap/1
  Switch1/1 -> Output_Range/1
  Add1/1 -> Switch2/1  "wrapPositionNegPii"
  Two_Pi2/1 -> Add1/2
  Switch2/1 -> Switch1/3
  Less_Than/1 -> Switch2/2  "positionLessThanPi"
  Add/1 -> Switch1/1  "wrapPositionPi"
  Two_Pi/1 -> Add/2
  Greater_Than/1 -> Switch1/2  "positionGreaterThanPii"
  Neg_Pi/1 -> Less_Than/2
  PI/1 -> Greater_Than/2
  Position/1 -> Input_Range/1

== system FieldOrientedController/EncoderToPositionAndVelocity/Rotor_To_Electrical_Position/Mod_Two_Pi ==
  note: Mod Two Pi
  X : Inport
  Mod : Math  Operator=mod  SignedPower=on  SaturateOnIntegerOverflow=on
  Two_Pi : Constant  Value=2*pi  OutDataTypeStr=Inherit: Inherit via back propagation
  Mod_X_Two_Pi : Outport  VectorParamsAs1DForOutWhenUnconnected=off
  wires:
  Mod/1 -> Mod_X_Two_Pi/1
  Two_Pi/1 -> Mod/2
  X/1 -> Mod/1

== system FieldOrientedController/Controller_Modes/Calibrate_Encoder_Offset/Encoder_Calibration/Count_To_Limit ==
  note: Count To Limit
  Reset : Inport
  Limit : Inport  Port=2
  Add : Sum
  Continue_Count : Constant  OutDataTypeStr=Inherit: Inherit via back propagation
  Delay : Delay  DelayLength=1  InitialCondition=0
  Delay1 : Delay  DelayLength=1  InitialCondition=0
  Greater_Or_Equal : RelationalOperator  OutDataTypeStr=boolean  RndMeth=Nearest
  Reset_Count : Constant  Value=0  OutDataTypeStr=Inherit: Inherit via back propagation
  Stop_Count : Constant  Value=0  OutDataTypeStr=Inherit: Inherit via back propagation
  Switch : Switch  Threshold=1
  Switch1 : Switch  Threshold=1
  At_Limit : Outport  VectorParamsAs1DForOutWhenUnconnected=off
  wires:
  Delay1/1 -> Switch1/2
  Limit/1 -> Greater_Or_Equal/2
  Switch1/1 -> Add/1
  Continue_Count/1 -> Switch1/3
  Switch/1 -> Delay/1, Greater_Or_Equal/1
  Stop_Count/1 -> Switch1/1
  Greater_Or_Equal/1 -> Delay1/1, At_Limit/1
  Delay/1 -> Add/2
  Reset/1 -> Switch/2
  Reset_Count/1 -> Switch/1
  Add/1 -> Switch/3

== system FieldOrientedController/Controller_Modes/Calibrate_Encoder_Offset/Encoder_Calibration/Negate_Zero_To_Two_Pi ==
  note: Negate Zero To Two Pi
  In : Inport
  Input_Range : SignalSpecification  OutMin=0  OutMax=2*pi
      settings: AttributesFormatString=|
      | -----------------------
      | Min = %<OutMin>
      | Max = %<OutMax>
  Subtract : Sum  Inputs=+-  OutDataTypeStr=Inherit: Inherit via back propagation
  Two_Pi : Constant  Value=2*pi  OutDataTypeStr=Inherit: Inherit via back propagation
  Out : Outport  VectorParamsAs1DForOutWhenUnconnected=off
  wires:
  Input_Range/1 -> Subtract/2
  Two_Pi/1 -> Subtract/1
  In/1 -> Input_Range/1
  Subtract/1 -> Out/1  "negativeIn"

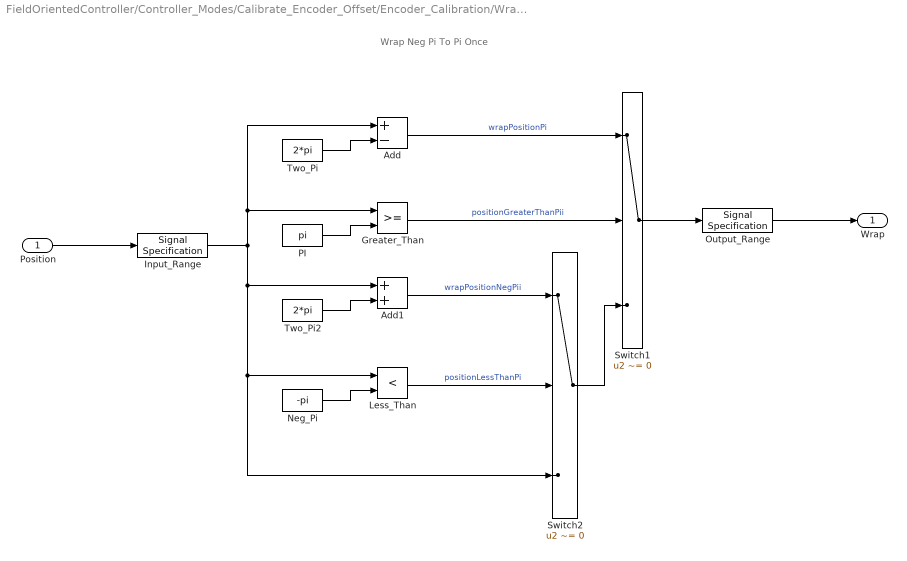
== system FieldOrientedController/Controller_Modes/Calibrate_Encoder_Offset/Encoder_Calibration/Wrap_Neg_Pi_To_Pi_Once ==
  note: Wrap Neg Pi To Pi Once
  Position : Inport
  Add : Sum  Inputs=+-  OutDataTypeStr=Inherit: Inherit via back propagation
  Add1 : Sum
  Greater_Than : RelationalOperator  OutDataTypeStr=boolean  RndMeth=Nearest
  Input_Range : SignalSpecification  OutMin=-4*pi  OutMax=4*pi
      settings: AttributesFormatString=|
      | -----------------------
      | Min = %<OutMin>
      | Max = %<OutMax>
  Less_Than : RelationalOperator  Operator=<  OutDataTypeStr=boolean  RndMeth=Nearest
  Neg_Pi : Constant  Value=-pi  OutDataTypeStr=Inherit: Inherit via back propagation
  Output_Range : SignalSpecification  OutMin=-pi  OutMax=pi
      settings: AttributesFormatString=|
      | -----------------------
      | Min = %<OutMin>
      | Max = %<OutMax>
  PI : Constant  Value=pi  OutDataTypeStr=Inherit: Inherit via back propagation
  Switch1 : Switch  Criteria=u2 ~= 0
  Switch2 : Switch  Criteria=u2 ~= 0
  Two_Pi : Constant  Value=2*pi  OutDataTypeStr=Inherit: Inherit via back propagation
  Two_Pi2 : Constant  Value=2*pi  OutDataTypeStr=Inherit: Inherit via back propagation
  Wrap : Outport  VectorParamsAs1DForOutWhenUnconnected=off
  wires:
  Input_Range/1 -> Greater_Than/1, Add/1, Add1/1, Switch2/3, Less_Than/1
  Output_Range/1 -> Wrap/1
  Switch1/1 -> Output_Range/1
  Add1/1 -> Switch2/1  "wrapPositionNegPii"
  Two_Pi2/1 -> Add1/2
  Switch2/1 -> Switch1/3
  Less_Than/1 -> Switch2/2  "positionLessThanPi"
  Add/1 -> Switch1/1  "wrapPositionPi"
  Two_Pi/1 -> Add/2
  Greater_Than/1 -> Switch1/2  "positionGreaterThanPii"
  Neg_Pi/1 -> Less_Than/2
  PI/1 -> Greater_Than/2
  Position/1 -> Input_Range/1

== system FieldOrientedController/Controller_Modes/Current_Control/FOC_Current_Control/Clarke_Transform ==
  note: Converts balanced three-phase quantities into balanced two-phase quantities.
      | The A and B phases are converted to the direct axis (alpha) component and the quadrature axis (beta) component.
      | The alpha and beta components are still dependent on time and speed.
  note: Clarke Transform
  ABC : Inport
  A : Selector  IndexMode=Zero-based  InputPortWidth=2  IndexOptions=Index vector (dialog)  Indices=0  OutputSizes=1
  Add : Sum  OutDataTypeStr=Inherit: Same as first input
  Alpha_Gain : Gain  Gain=1/sqrt(3)
  B : Selector  IndexMode=Zero-based  InputPortWidth=2  IndexOptions=Index vector (dialog)  Indices=1  OutputSizes=1
  Beta_Gain : Gain  Gain=2/sqrt(3)
  Alpha : Outport  VectorParamsAs1DForOutWhenUnconnected=off
  Beta : Outport  Port=2  VectorParamsAs1DForOutWhenUnconnected=off
  wires:
  A/1 -> Alpha/1, Alpha_Gain/1
  Alpha_Gain/1 -> Add/1
  ABC/1 -> B/1, A/1
  Beta_Gain/1 -> Add/2
  B/1 -> Beta_Gain/1
  Add/1 -> Beta/1

== system FieldOrientedController/Controller_Modes/Current_Control/FOC_Current_Control/DQ_Current_Control ==
  note: DQ Current Control
  Q_Command : Inport
  D_Current : Inport  Port=2
  Q_Current : Inport  Port=3
  D_Command : Constant  Value=0  OutDataTypeStr=Inherit: Inherit via back propagation
  D_Current_Control : Subsystem
  Q_Current_Control : Subsystem
  D_Voltage : Outport  VectorParamsAs1DForOutWhenUnconnected=off
  Q_Voltage : Outport  Port=2  VectorParamsAs1DForOutWhenUnconnected=off
  wires:
  D_Current/1 -> D_Current_Control/2(Current_Measured)
  Q_Current/1 -> Q_Current_Control/2(Current_Measured)
  D_Current_Control/1(Voltage) -> D_Voltage/1
  Q_Current_Control/1(Voltage) -> Q_Voltage/1
  Q_Command/1 -> Q_Current_Control/1(Current_Command)
  D_Command/1 -> D_Current_Control/1(Current_Command)

== system FieldOrientedController/Controller_Modes/Current_Control/FOC_Current_Control/Inverse_Clarke_Transform ==
  note: Inverse Clarke Transform
  note: Converts direct axis (alpha) component and the quadrature axis (beta) component to balanced three-phase quantities
      | The alpha and beta components are dependent on time and speed.
  Alpha : Inport
  Beta : Inport  Port=2
  Add : Sum  Inputs=-+  OutDataTypeStr=Inherit: Same as first input
  Add1 : Sum  Inputs=--  OutDataTypeStr=Inherit: Same as first input
  Gain : Gain  Gain=1/2
  Gain1 : Gain  Gain=sqrt(3)/2
  a : Outport  VectorParamsAs1DForOutWhenUnconnected=off
  b : Outport  Port=2  VectorParamsAs1DForOutWhenUnconnected=off
  b1 : Outport  Port=3  VectorParamsAs1DForOutWhenUnconnected=off
  wires:
  Gain/1 -> Add1/1, Add/1
  Gain1/1 -> Add1/2, Add/2
  Add/1 -> b/1
  Add1/1 -> b1/1
  Beta/1 -> Gain1/1
  Alpha/1 -> a/1, Gain/1

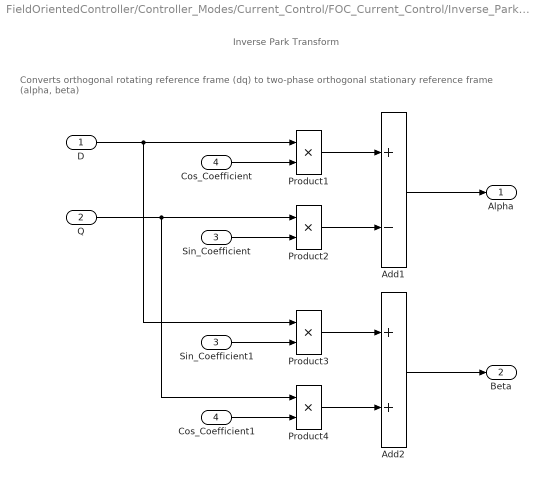
== system FieldOrientedController/Controller_Modes/Current_Control/FOC_Current_Control/Inverse_Park_Transform ==
  note: Inverse Park Transform
  note: Converts orthogonal rotating reference frame (dq) to two-phase orthogonal stationary reference frame (alpha, beta)
  D : Inport
  Q : Inport  Port=2
  Sin_Coefficient : Inport  Port=3
  Cos_Coefficient : Inport  Port=4
  Add1 : Sum  Inputs=+-  OutDataTypeStr=Inherit: Same as first input
  Add2 : Sum  OutDataTypeStr=Inherit: Same as first input
  Cos_Coefficient1 : InportShadow  Port=4
  Product{1..4} (4 alike) : Product  RndMeth=Simplest
  Sin_Coefficient1 : InportShadow  Port=3
  Alpha : Outport  VectorParamsAs1DForOutWhenUnconnected=off
  Beta : Outport  Port=2  VectorParamsAs1DForOutWhenUnconnected=off
  wires:
  Add2/1 -> Beta/1
  Add1/1 -> Alpha/1
  Product3/1 -> Add2/1
  Product4/1 -> Add2/2
  Product1/1 -> Add1/1
  Product2/1 -> Add1/2
  Cos_Coefficient1/1 -> Product4/2
  Sin_Coefficient/1 -> Product2/2
  D/1 -> Product3/1, Product1/1
  Q/1 -> Product2/1, Product4/1
  Sin_Coefficient1/1 -> Product3/2
  Cos_Coefficient/1 -> Product1/2

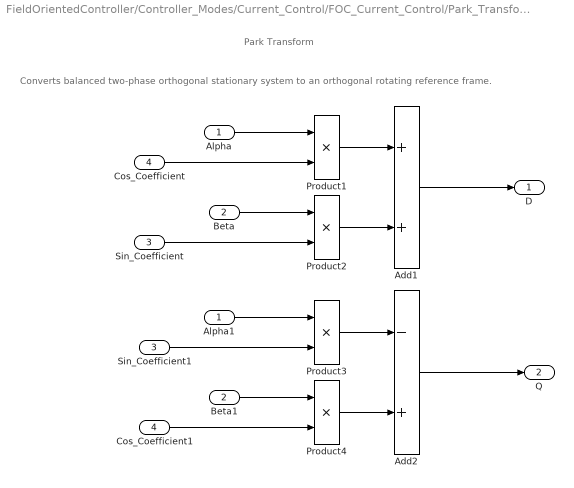
== system FieldOrientedController/Controller_Modes/Current_Control/FOC_Current_Control/Park_Transform ==
  note: Converts balanced two-phase orthogonal stationary system to an orthogonal rotating reference frame.
  note: Park Transform
  Alpha : Inport
  Beta : Inport  Port=2
  Sin_Coefficient : Inport  Port=3
  Cos_Coefficient : Inport  Port=4
  Add1 : Sum  OutDataTypeStr=Inherit: Same as first input
  Add2 : Sum  Inputs=-+  OutDataTypeStr=Inherit: Same as first input
  Alpha1 : InportShadow
  Beta1 : InportShadow  Port=2
  Cos_Coefficient1 : InportShadow  Port=4
  Product{1..4} (4 alike) : Product  RndMeth=Simplest
  Sin_Coefficient1 : InportShadow  Port=3
  D : Outport  VectorParamsAs1DForOutWhenUnconnected=off
  Q : Outport  Port=2  VectorParamsAs1DForOutWhenUnconnected=off
  wires:
  Add2/1 -> Q/1
  Add1/1 -> D/1
  Sin_Coefficient/1 -> Product2/2
  Beta/1 -> Product2/1
  Cos_Coefficient/1 -> Product1/2
  Alpha/1 -> Product1/1
  Beta1/1 -> Product4/1
  Cos_Coefficient1/1 -> Product4/2
  Sin_Coefficient1/1 -> Product3/2
  Alpha1/1 -> Product3/1
  Product2/1 -> Add1/2
  Product1/1 -> Add1/1
  Product4/1 -> Add2/2
  Product3/1 -> Add2/1

== system FieldOrientedController/Controller_Modes/Current_Control/FOC_Current_Control/Space_Vector_Modulation1 ==
  note: Space Vector Modulation
  ABC : Inport
  Add : Sum
  Add1 : Sum  Inputs=+-
  Gain : Gain  Gain=0.5  OutDataTypeStr=Inherit: Same as input
  Max : MinMax  Function=max
  Min : MinMax
  ABC_SVM : Outport  VectorParamsAs1DForOutWhenUnconnected=off
  wires:
  Add/1 -> Gain/1
  Max/1 -> Add/1
  Min/1 -> Add/2
  Gain/1 -> Add1/2
  ABC/1 -> Add1/1, Max/1, Min/1
  Add1/1 -> ABC_SVM/1

== system FieldOrientedController/Controller_Modes/Open_Loop_Velocity_Control/Open_Loop_Velocity_Control/Electrical_Velocity_To_Position ==
  note: Electrical Velocity To Position
  EV : Inport
  Add : Sum
  Delay : Delay  DelayLength=1
  Gain : Gain  Gain=sampleTime.OpenLoopVelocityControl  OutDataTypeStr=Inherit: Inherit via back propagation
      settings: AttributesFormatString=------------------------------\nGain = %<Gain>
  Mod_Two_Pi_Once : Subsystem
      mask Display:
      | text(0.5, 0.5,'Mod 2\pi',...
      |   'HorizontalAlignment', 'Center',...
      |   'VerticalAlignment', 'Middle',...
      |   'texmode', 'on')
  EP : Outport  VectorParamsAs1DForOutWhenUnconnected=off
  wires:
  Add/1 -> Mod_Two_Pi_Once/1(X)
  Mod_Two_Pi_Once/1(Mod_X_Two_Pi) -> Delay/1
  EV/1 -> Gain/1
  Gain/1 -> Add/1
  Delay/1 -> EP/1, Add/2

== system FieldOrientedController/Controller_Modes/Open_Loop_Velocity_Control/Open_Loop_Velocity_Control/Inverse_Clarke_Transform1 ==
  note: Inverse Clarke Transform
  note: Converts direct axis (alpha) component and the quadrature axis (beta) component to balanced three-phase quantities
      | The alpha and beta components are dependent on time and speed.
  Alpha : Inport
  Beta : Inport  Port=2
  Add : Sum  Inputs=-+  OutDataTypeStr=Inherit: Same as first input
  Add1 : Sum  Inputs=--  OutDataTypeStr=Inherit: Same as first input
  Gain : Gain  Gain=1/2
  Gain1 : Gain  Gain=sqrt(3)/2
  a : Outport  VectorParamsAs1DForOutWhenUnconnected=off
  b : Outport  Port=2  VectorParamsAs1DForOutWhenUnconnected=off
  b1 : Outport  Port=3  VectorParamsAs1DForOutWhenUnconnected=off
  wires:
  Gain/1 -> Add1/1, Add/1
  Gain1/1 -> Add1/2, Add/2
  Add/1 -> b/1
  Add1/1 -> b1/1
  Beta/1 -> Gain1/1
  Alpha/1 -> a/1, Gain/1

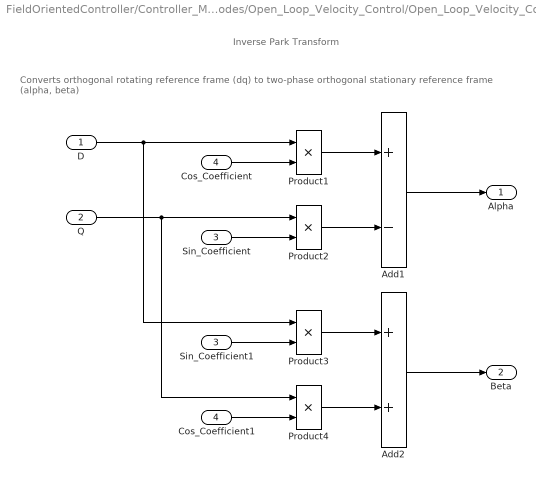
== system FieldOrientedController/Controller_Modes/Open_Loop_Velocity_Control/Open_Loop_Velocity_Control/Inverse_Park_Transform ==
  note: Inverse Park Transform
  note: Converts orthogonal rotating reference frame (dq) to two-phase orthogonal stationary reference frame (alpha, beta)
  D : Inport
  Q : Inport  Port=2
  Sin_Coefficient : Inport  Port=3
  Cos_Coefficient : Inport  Port=4
  Add1 : Sum  Inputs=+-  OutDataTypeStr=Inherit: Same as first input
  Add2 : Sum  OutDataTypeStr=Inherit: Same as first input
  Cos_Coefficient1 : InportShadow  Port=4
  Product{1..4} (4 alike) : Product  RndMeth=Simplest
  Sin_Coefficient1 : InportShadow  Port=3
  Alpha : Outport  VectorParamsAs1DForOutWhenUnconnected=off
  Beta : Outport  Port=2  VectorParamsAs1DForOutWhenUnconnected=off
  wires:
  Add2/1 -> Beta/1
  Add1/1 -> Alpha/1
  Product3/1 -> Add2/1
  Product4/1 -> Add2/2
  Product1/1 -> Add1/1
  Product2/1 -> Add1/2
  Cos_Coefficient1/1 -> Product4/2
  Sin_Coefficient/1 -> Product2/2
  D/1 -> Product3/1, Product1/1
  Q/1 -> Product2/1, Product4/1
  Sin_Coefficient1/1 -> Product3/2
  Cos_Coefficient/1 -> Product1/2

== system FieldOrientedController/Controller_Modes/Open_Loop_Velocity_Control/Open_Loop_Velocity_Control/Ramp_Velocity ==
  note: Ramp Velocity
  Velocity_Command : Inport
  Delay : Delay  DelayLength=1
  Gain : Gain  Gain=sampleTime.OpenLoopVelocityControl  OutDataTypeStr=Inherit: Same as input
      settings: AttributesFormatString=------------------------------\nGain = %<Gain>
  Number_Of_Pole_Pairs : Gain  Gain=PolePairs
      settings: AttributesFormatString=------------------------------------\nGain = %<Gain>
  Set_Acceleration : Subsystem
  Sum : Sum  Inputs=++|  SaturateOnIntegerOverflow=on
  Rotor_Velocity : Outport  VectorParamsAs1DForOutWhenUnconnected=off
  Electrical_Velocity : Outport  Port=2  VectorParamsAs1DForOutWhenUnconnected=off
  wires:
  Sum/1 -> Delay/1
  Delay/1 -> Rotor_Velocity/1, Number_Of_Pole_Pairs/1, Sum/2, Set_Acceleration/2(V_Current)
  Gain/1 -> Sum/1
  Velocity_Command/1 -> Set_Acceleration/1(V_Target)
  Set_Acceleration/1(A) -> Gain/1
  Number_Of_Pole_Pairs/1 -> Electrical_Velocity/1

== system FieldOrientedController/Controller_Modes/Open_Loop_Velocity_Control/Open_Loop_Velocity_Control/Rotor_Velocity_To_Volts ==
  note: Rotor Velocity To Volts
  RV : Inport
  Abs : Abs
  Add : Sum  OutDataTypeStr=Inherit: Same as first input
  Frequency_To_Voltage : Gain  Gain=paramOpenLoopVelocityToVoltsScalar
      settings: AttributesFormatString=--------------------------------\n%<Gain>
  Voltage_Bias : Constant  Value=paramOpenLoopVelocityToVoltsBias  OutDataTypeStr=Inherit: Inherit via back propagation  SampleTime=-1
  V : Outport  VectorParamsAs1DForOutWhenUnconnected=off
  wires:
  Voltage_Bias/1 -> Add/1
  Add/1 -> V/1
  Frequency_To_Voltage/1 -> Add/2
  Abs/1 -> Frequency_To_Voltage/1
  RV/1 -> Abs/1
